simulink model "Dyn_Vol_Line"  (R2019b)
settings: Solver=ode4  StartTime=0.0  StopTime=5  FixedStep=0.0005  MaxStep=0.1  RelTol=1e-3  EnableMultiTasking=on
undefined symbols (not defined in the file): H2
libraries: Lib_Vol_pipeCd_TMATS x4, Lib_Vol_Volume_TMATS x4, Lib_Solve_ModelSource_TMATS x2, Lib_Vol_Valve_TMATS x2, Lib_Solve_IterNRSolverJC_TMATS x1, Lib_Vol_FlowChar_TMATS x1, Lib_Vol_FlowStart_TMATS x1, Lib_Vol_PropLookup_TMATS x1
settings Model: SimulationMode=rapid-accelerator  Creator=jwchapm2  LastModifiedBy=bhisma
settings DataIOCC: LimitDataPoints=on  SaveFormat=Array  ReturnWorkspaceOutputs=off
settings OptimizationCC: LifeSpan=inf
settings DebuggingCC: SFUnexpectedBacktrackingDiag=warning  SFNoUnconditionalDefaultTransitionDiag=warning  SFExecutionAtInitializationDiag=none  ArithmeticOperatorsInVariantConditions=warning
settings HardwareCC: ProdBitPerPointer=32  ProdBitPerSizeT=32  ProdBitPerPtrDiffT=32  ProdLargestAtomicFloat=None  ProdIntDivRoundTo=Undefined  ProdEndianess=Unspecified  ProdWordSize=32  ProdHWDeviceType=32-bit Generic
settings ModelReferenceCC: PropagateSignalLabelsOutOfModel=off
settings SFSimCC: SimUseLocalCustomCode=off  CustomCodeUndefinedFunction=UseInterfaceOnly
settings RTWCC: RTWUseLocalCustomCode=off
settings CodeAppCC: StateflowObjectComments=on
settings GRTTargetCC: TargetLangStandard=C89/C90 (ANSI)  GeneratePreprocessorConditionals=Disable all
settings ConfigComp: CovMetricSettings=dw  CovHtmlReporting=on  CovSaveCumulativeToWorkspaceVar=on  CovSaveSingleToWorkspaceVar=on  CovExternalEMLEnable=off

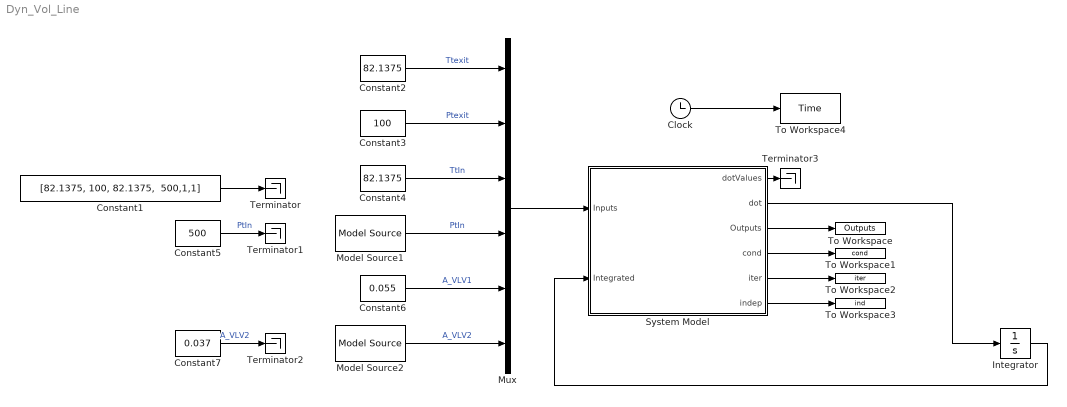
== system Dyn_Vol_Line ==
  Clock : Clock
  Constant1 : Constant  Value="[82.1375, 100, 82.1375,  500,1,1]"
  Constant2 : Constant  Value=82.1375
  Constant3 : Constant  Value=100
  Constant4 : Constant  Value=82.1375
  Constant5 : Constant  Value=500
  Constant6 : Constant  Value=0.055
  Constant7 : Constant  Value=0.037
  Integrator : Integrator  InitialCondition=[1.656, 47.38, 1.234, 52.46, 1.226, 52.55, 1.059, 54.12]
  Model Source1 : Lib_Solve_ModelSource_TMATS/Model Source  T_vec_M=[0 0.1 5]  input_array_M=[500 1000 50]
  Model Source2 : Lib_Solve_ModelSource_TMATS/Model Source  T_vec_M=[0 0.1 3 5]  input_array_M=[0.037 0.037 0 0 ]
  Mux : Mux  Inputs=6
  System Model : Subsystem
  Terminator{,1..3} (4 alike) : Terminator
  To Workspace : ToWorkspace  VariableName=Outputs  SampleTime=-1
      settings: Save2DSignal=2-D array (concatenate along first dimension)
  To Workspace1 : ToWorkspace  VariableName=cond  SampleTime=-1
      settings: Save2DSignal=2-D array (concatenate along first dimension)
  To Workspace2 : ToWorkspace  VariableName=iter  SampleTime=-1
      settings: Save2DSignal=2-D array (concatenate along first dimension)
  To Workspace3 : ToWorkspace  VariableName=ind  SampleTime=-1
      settings: Save2DSignal=2-D array (concatenate along first dimension)
  To Workspace4 : ToWorkspace  VariableName=Time  SampleTime=-1
      settings: Save2DSignal=2-D array (concatenate along first dimension)
  wires:
  Mux/1 -> System Model/1(Inputs)
  Integrator/1 -> System Model/2(Integrated)
  System Model/2(dot) -> Integrator/1
  Constant2/1 -> Mux/1  "Ttexit"
  Constant3/1 -> Mux/2  "Ptexit"
  Constant4/1 -> Mux/3  "TtIn"
  Model Source1/1 -> Mux/4  "PtIn"
  Constant6/1 -> Mux/5  "A_VLV1"
  Model Source2/1 -> Mux/6  "A_VLV2"
  System Model/3(Outputs) -> To Workspace/1
  System Model/4(cond) -> To Workspace1/1
  System Model/5(iter) -> To Workspace2/1
  System Model/6(indep) -> To Workspace3/1
  Clock/1 -> To Workspace4/1
  Constant1/1 -> Terminator/1
  Constant5/1 -> Terminator1/1  "PtIn"
  Constant7/1 -> Terminator2/1  "A_VLV2"
  System Model/1(dotValues) -> Terminator3/1

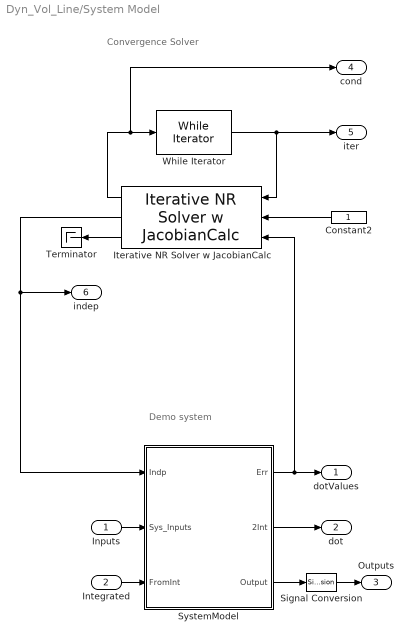
== system Dyn_Vol_Line/System Model ==
  note: Convergence Solver
  note: Demo system
  Inputs : Inport
  Integrated : Inport  Port=2
  Constant2 : Constant
  Iterative NR Solver w JacobianCalc : Lib_Solve_IterNRSolverJC_TMATS/Iterative NR Solver w JacobianCalc  SJac_Per_M=[0.05* ones(8,1)';-0.05* ones(8,1)']  SNR_IC_M=[453.3 98.05 303.8 98.05 301.2 98.05 251.1 98.05]  SNR_DX_M=1  SNR_Mx_M=100000  SNR_Mn_M=0.0001  SJacobianAttempts_M=50  Cond_Limits_M=0.00000001
  Signal Conversion : SignalConversion  OverrideOpt=off
  SystemModel : Subsystem  mask{Fluid=H2}
      mask prompts: Fluid "Fluid Type"
  Terminator : Terminator
  While Iterator : WhileIterator  MaxIters=200  WhileBlockType=do-while  ShowIterationPort=on
  dotValues : Outport
  dot : Outport  Port=2
  Outputs : Outport  Port=3
  cond : Outport  Port=4
  iter : Outport  Port=5
  indep : Outport  Port=6
  wires:
  Constant2/1 -> Iterative NR Solver w JacobianCalc/2
  Inputs/1 -> SystemModel/2(Sys_Inputs)
  SystemModel/1(Err) -> dotValues/1, Iterative NR Solver w JacobianCalc/3
  Iterative NR Solver w JacobianCalc/2 -> indep/1, SystemModel/1(Indp)
  SystemModel/2(2Int) -> dot/1
  Integrated/1 -> SystemModel/3(FromInt)
  Iterative NR Solver w JacobianCalc/1 -> cond/1, While Iterator/1
  While Iterator/1 -> iter/1, Iterative NR Solver w JacobianCalc/1
  Iterative NR Solver w JacobianCalc/3 -> Terminator/1
  SystemModel/3(Output) -> Signal Conversion/1
  Signal Conversion/1 -> Outputs/1

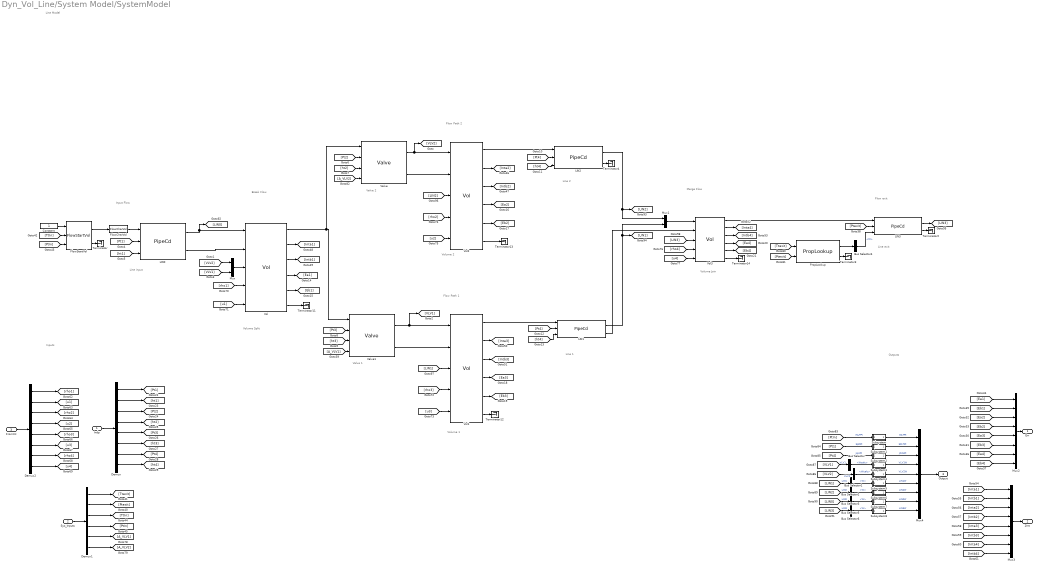
== system Dyn_Vol_Line/System Model/SystemModel ==
  note: Line Model
  note: Flow Path 2
  note: Flow Path 1
  note: Valve 2
  note: Valve 1
  note: Volume 1
  note: Line 1
  note: Volume 2
  note: Line 2
  note: Volume
      | Join
  note: Flow exit
  note: Merge
      | Flow
  note: Break
      | Flow
  note: Volume
      | Split
  note: Input Flow
  note: Line exit
  note: Inputs
  note: Outputs
  note: Line input
  Indp : Inport
  Sys_Inputs : Inport  Port=2
  FromInt : Inport  Port=3
  Bus Selector : BusSelector  OutputSignals=Wcalc
  Bus Selector1 : BusSelector  OutputSignals=Wcalc
  Bus Selector{2..3,5..6} (4 alike) : BusSelector  OutputSignals=W
  Bus Selector4 : BusSelector  OutputSignals=ht
  Constant : Constant
  Demux : Demux  Outputs=8
  Demux1 : Demux  Outputs=6
  Demux2 : Demux  Outputs=8
  FlowCharVol : Lib_Vol_FlowChar_TMATS/FlowCharVol  SystemSampleTime=-1
  FlowStartVol : Lib_Vol_FlowStart_TMATS/FlowStartVol  TtVec_M=Fluid.Vec.Tt  PtVec_M=Fluid.Vec.Pt  htVec_M=Fluid.Vec.ht  sVec_M=Fluid.Vec.s  htArray_M=Fluid.Array.ht  TtArray_M=Fluid.Array.Tt  sArray_M=Fluid.Array.s  rhoArray_M=Fluid.Array.rho  muArray_M=Fluid.Array.mu  CpArray_M=Fluid.Array.Cp  CvArray_M=Fluid.Array.Cv  CvArray_M_copy=Fluid.Array.u  Rval_M=Fluid.Array.R
  LIN0 : Lib_Vol_pipeCd_TMATS/PipeCd  Cd_M=0.5541  A_M=1  htVec_M=Fluid.Vec.ht  PtVec_M=Fluid.Vec.Pt  TtArray_M=Fluid.Array.Tt  rhoArray_M=Fluid.Array.rho
  LIN1 : Lib_Vol_pipeCd_TMATS/PipeCd  Cd_M=0.3859  A_M=1  htVec_M=Fluid.Vec.ht  PtVec_M=Fluid.Vec.Pt  TtArray_M=Fluid.Array.Tt  rhoArray_M=Fluid.Array.rho
  LIN2 : Lib_Vol_pipeCd_TMATS/PipeCd  Cd_M=0.2502  A_M=1  htVec_M=Fluid.Vec.ht  PtVec_M=Fluid.Vec.Pt  TtArray_M=Fluid.Array.Tt  rhoArray_M=Fluid.Array.rho
  LIN3 : Lib_Vol_pipeCd_TMATS/PipeCd  Cd_M=0.3985  A_M=1  htVec_M=Fluid.Vec.ht  PtVec_M=Fluid.Vec.Pt  TtArray_M=Fluid.Array.Tt  rhoArray_M=Fluid.Array.rho
  Mux : Mux  Inputs=2
  Mux1 : Mux  Inputs=2
  Mux2 : Mux  Inputs=8
  Mux3 : Mux  Inputs=8
  Mux4 : Mux  Inputs=9
  PropLookup : Lib_Vol_PropLookup_TMATS/PropLookup  case_M='ht'  propg_M=0  htg_M=0  htVec_M=Fluid.Vec.ht  PtVec_M=Fluid.Vec.Pt  TtVec_M=[-10000 10000]  sVec_M=[-10000 10000]  htArray_M=ones(2, length(Fluid.Vec.Pt))'  rhoArray_M=ones(length(Fluid.Vec.ht), length(Fluid.Vec.Pt))'  uArray_M=ones(length(Fluid.Vec.ht), length(Fluid.Vec.Pt))'  sArray_M=ones(length(Fluid.Vec.ht), length(Fluid.Vec.Pt))'  muArray_M=ones(length(Fluid.Vec.ht), length(Fluid.Vec.Pt))'  ThArray_M=Fluid.Array.Tt  CvArray_M=ones(length(Fluid.Vec.ht), length(Fluid.Vec.Pt))'  CpArray_M=ones(length(Fluid.Vec.ht), length(Fluid.Vec.Pt))'  kArray_M=ones(length(Fluid.Vec.ht), length(Fluid.Vec.Pt))'  TsArray_M=ones(2, length(Fluid.Vec.Pt))'  hsArray_M=ones(2, length(Fluid.Vec.Pt))'  Rval_M=0
  Subsystem : Subsystem
  Subsystem1 : Subsystem
  Subsystem2 : Subsystem
  Subsystem3 : Subsystem
  Subsystem4 : Subsystem
  Subsystem5 : Subsystem
  Subsystem6 : Subsystem
  Subsystem7 : Subsystem
  Subsystem8 : Subsystem
  Terminator{,2..4,11..14} (8 alike) : Terminator
  Valve : Lib_Vol_Valve_TMATS/Valve  Cd_M=3.4641  htVec_M=Fluid.Vec.ht  PtVec_M=Fluid.Vec.Pt  TtArray_M=Fluid.Array.Tt  rhoArray_M=Fluid.Array.rho
  Valve1 : Lib_Vol_Valve_TMATS/Valve  Cd_M=3.4641  htVec_M=Fluid.Vec.ht  PtVec_M=Fluid.Vec.Pt  TtArray_M=Fluid.Array.Tt  rhoArray_M=Fluid.Array.rho
  Vol : Lib_Vol_Volume_TMATS/Vol  volume_M=300  htVec_M=Fluid.Vec.ht  PtVec_M=Fluid.Vec.Pt  TtArray_M=Fluid.Array.Tt  uArray_M=Fluid.Array.u  rhoArray_M=Fluid.Array.rho
  Vol1 : Lib_Vol_Volume_TMATS/Vol  volume_M=1000  htVec_M=Fluid.Vec.ht  PtVec_M=Fluid.Vec.Pt  TtArray_M=Fluid.Array.Tt  uArray_M=Fluid.Array.u  rhoArray_M=Fluid.Array.rho
  Vol2 : Lib_Vol_Volume_TMATS/Vol  volume_M=500  htVec_M=Fluid.Vec.ht  PtVec_M=Fluid.Vec.Pt  TtArray_M=Fluid.Array.Tt  uArray_M=Fluid.Array.u  rhoArray_M=Fluid.Array.rho
  Vol3 : Lib_Vol_Volume_TMATS/Vol  volume_M=500  htVec_M=Fluid.Vec.ht  PtVec_M=Fluid.Vec.Pt  TtArray_M=Fluid.Array.Tt  uArray_M=Fluid.Array.u  rhoArray_M=Fluid.Array.rho
  Err : Outport
  2Int : Outport  Port=2
  Output : Outport  Port=3
  wires:
  Vol2/3 -> [Intb2]
  LIN3/2 -> Terminator2/1
  Bus Selector4/1 -> LIN3/3  "<ht>"
  [Ptexit] -> LIN3/2
  FlowStartVol/1 -> FlowCharVol/1
  FlowStartVol/2 -> Terminator/1
  LIN0/2 -> Vol/2
  Mux/1 -> Vol/3
  Valve/2 -> Vol2/2
  Valve1/2 -> Vol1/2
  Mux1/1 -> Vol3/1
  LIN1/2 -> Vol3/2
  [VLV2] -> Mux/1
  [VLV1] -> Mux/2
  [Pt1] -> LIN0/2
  [ht1] -> LIN0/3
  [ht2] -> Valve/3
  [Pt3] -> Valve1/2
  [ht3] -> Valve1/3
  [Pt4] -> LIN2/2
  [ht4] -> LIN2/3
  [ht4] -> LIN1/3
  Vol/4 -> [Ea1]
  Vol/5 -> [Eb1]
  Vol2/4 -> [Ea2]
  Vol2/5 -> [Eb2]
  Vol1/4 -> [Ea3]
  Vol1/5 -> [Eb3]
  Vol3/4 -> [Ea4]
  Vol3/5 -> [Eb4]
  Constant/1 -> FlowStartVol/1
  Mux2/1 -> Err/1
  Indp/1 -> Demux/1
  Vol2/2 -> [Inta2]
  [TtIn] -> FlowStartVol/2
  [Ea1] -> Mux2/1
  [Ea3] -> Mux2/5
  [Eb1] -> Mux2/2
  Demux/8 -> [ht4]
  Demux/5 -> [Pt3]
  Demux/2 -> [ht1]
  Demux/6 -> [ht3]
  [PtIn] -> FlowStartVol/3
  Demux/3 -> [Pt2]
  [Eb2] -> Mux2/4
  [Ea4] -> Mux2/7
  Demux/1 -> [Pt1]
  [Eb3] -> Mux2/6
  [Eb4] -> Mux2/8
  Demux/7 -> [Pt4]
  Demux/4 -> [ht2]
  [Ea2] -> Mux2/3
  Demux1/4 -> [PtIn]
  Demux1/3 -> [TtIn]
  Demux1/2 -> [Ptexit]
  Demux1/1 -> [Ttexit]
  Sys_Inputs/1 -> Demux1/1
  FlowCharVol/1 -> LIN0/1
  Vol1/1 -> LIN1/1
  Vol2/1 -> LIN2/1
  Vol3/1 -> LIN3/1
  LIN2/1 -> [LIN2], Mux1/1
  LIN1/1 -> [LIN1], Mux1/2
  LIN3/1 -> [LIN3]
  Valve/1 -> Vol2/1, [VLV2]
  Valve1/1 -> Vol1/1, [VLV1]
  LIN0/1 -> Vol/1, [LIN0]
  [Pt4] -> LIN1/2
  Vol/6 -> Terminator11/1
  Vol1/2 -> [Inta3]
  Vol1/3 -> [Intb3]
  Vol1/6 -> Terminator12/1
  Vol2/6 -> Terminator13/1
  Vol3/6 -> Terminator14/1
  Vol3/3 -> [Intb4]
  Vol3/2 -> [Inta4]
  Vol/2 -> [Inta1]
  Vol/3 -> [Intb1]
  [Inta3] -> Mux3/5
  [Intb2] -> Mux3/4
  [Intb3] -> Mux3/6
  [Inta4] -> Mux3/7
  [Inta2] -> Mux3/3
  [Intb1] -> Mux3/2
  [Intb4] -> Mux3/8
  [Inta1] -> Mux3/1
  Mux3/1 -> 2Int/1
  FromInt/1 -> Demux2/1
  Demux2/1 -> [rho1]
  Demux2/2 -> [u1]
  Demux2/3 -> [rho2]
  Demux2/4 -> [u2]
  Demux2/5 -> [rho3]
  Demux2/6 -> [u3]
  Demux2/7 -> [rho4]
  Demux2/8 -> [u4]
  [u1] -> Vol/5
  [rho1] -> Vol/4
  [rho3] -> Vol1/4
  [u3] -> Vol1/5
  [rho2] -> Vol2/4
  [u2] -> Vol2/5
  [rho4] -> Vol3/4
  [u4] -> Vol3/5
  Demux1/5 -> [A_VLV1]
  Demux1/6 -> [A_VLV2]
  [Ttexit] -> PropLookup/1
  [Ptexit] -> PropLookup/2
  PropLookup/1 -> Bus Selector4/1
  PropLookup/2 -> Terminator3/1
  [A_VLV2] -> Valve/4
  [A_VLV1] -> Valve1/4
  [VLV1] -> Bus Selector/1  "VLV1"
  [VLV2] -> Bus Selector1/1  "VLV2"
  [LIN1] -> Bus Selector2/1  "LIN1"
  [LIN2] -> Bus Selector3/1  "LIN2"
  [LIN0] -> Bus Selector5/1  "LIN0"
  [LIN3] -> Bus Selector6/1  "LIN3"
  [PtIn] -> Subsystem/1(In1)  "INLTPt"
  [Pt1] -> Subsystem1/1(In1)  "SpltPt"
  [Pt4] -> Subsystem2/1(In1)  "JoinPt"
  Bus Selector/1 -> Subsystem3/1(In1)  "<Wcalc>"
  Bus Selector1/1 -> Subsystem4/1(In1)  "<Wcalc>"
  Bus Selector2/1 -> Subsystem5/1(In1)  "<W>"
  Bus Selector3/1 -> Subsystem6/1(In1)  "<W>"
  Bus Selector5/1 -> Subsystem7/1(In1)  "<W>"
  Bus Selector6/1 -> Subsystem8/1(In1)  "<W>"
  Mux4/1 -> Output/1
  Subsystem/1(Out1) -> Mux4/1  "INLTPt"
  Subsystem1/1(Out1) -> Mux4/2  "SPLTPt"
  Subsystem2/1(Out1) -> Mux4/3  "JOINPt"
  Subsystem3/1(Out1) -> Mux4/4  "VLV1W"
  Subsystem4/1(Out1) -> Mux4/5  "VLV2W"
  Subsystem5/1(Out1) -> Mux4/6  "LIN1W"
  Subsystem6/1(Out1) -> Mux4/7  "LIN2W"
  Subsystem7/1(Out1) -> Mux4/8  "LIN0W"
  Subsystem8/1(Out1) -> Mux4/9  "LIN3W"
  LIN2/2 -> Terminator4/1
  [LIN2] -> Vol2/3
  [LIN1] -> Vol1/3
  [LIN3] -> Vol3/3
  Vol/1 -> Valve1/1, Valve/1
  [Pt2] -> Valve/2

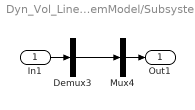
== system Dyn_Vol_Line/System Model/SystemModel/Subsystem ==
  In1 : Inport
  Demux3 : Demux  Outputs=1
  Mux4 : Mux  Inputs=1
  Out1 : Outport
  wires:
  Demux3/1 -> Mux4/1
  In1/1 -> Demux3/1
  Mux4/1 -> Out1/1

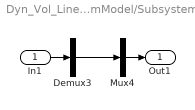
== system Dyn_Vol_Line/System Model/SystemModel/Subsystem1 ==
  In1 : Inport
  Demux3 : Demux  Outputs=1
  Mux4 : Mux  Inputs=1
  Out1 : Outport
  wires:
  Mux4/1 -> Out1/1
  In1/1 -> Demux3/1
  Demux3/1 -> Mux4/1

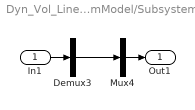
== system Dyn_Vol_Line/System Model/SystemModel/Subsystem2 ==
  In1 : Inport
  Demux3 : Demux  Outputs=1
  Mux4 : Mux  Inputs=1
  Out1 : Outport
  wires:
  Demux3/1 -> Mux4/1
  In1/1 -> Demux3/1
  Mux4/1 -> Out1/1

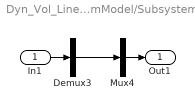
== system Dyn_Vol_Line/System Model/SystemModel/Subsystem3 ==
  In1 : Inport
  Demux3 : Demux  Outputs=1
  Mux4 : Mux  Inputs=1
  Out1 : Outport
  wires:
  Mux4/1 -> Out1/1
  In1/1 -> Demux3/1
  Demux3/1 -> Mux4/1

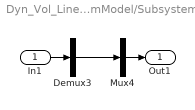
== system Dyn_Vol_Line/System Model/SystemModel/Subsystem4 ==
  In1 : Inport
  Demux3 : Demux  Outputs=1
  Mux4 : Mux  Inputs=1
  Out1 : Outport
  wires:
  Demux3/1 -> Mux4/1
  In1/1 -> Demux3/1
  Mux4/1 -> Out1/1

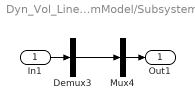
== system Dyn_Vol_Line/System Model/SystemModel/Subsystem5 ==
  In1 : Inport
  Demux3 : Demux  Outputs=1
  Mux4 : Mux  Inputs=1
  Out1 : Outport
  wires:
  Mux4/1 -> Out1/1
  In1/1 -> Demux3/1
  Demux3/1 -> Mux4/1

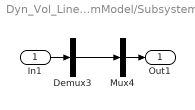
== system Dyn_Vol_Line/System Model/SystemModel/Subsystem6 ==
  In1 : Inport
  Demux3 : Demux  Outputs=1
  Mux4 : Mux  Inputs=1
  Out1 : Outport
  wires:
  Demux3/1 -> Mux4/1
  In1/1 -> Demux3/1
  Mux4/1 -> Out1/1

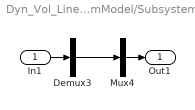
== system Dyn_Vol_Line/System Model/SystemModel/Subsystem7 ==
  In1 : Inport
  Demux3 : Demux  Outputs=1
  Mux4 : Mux  Inputs=1
  Out1 : Outport
  wires:
  Mux4/1 -> Out1/1
  In1/1 -> Demux3/1
  Demux3/1 -> Mux4/1

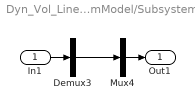
== system Dyn_Vol_Line/System Model/SystemModel/Subsystem8 ==
  In1 : Inport
  Demux3 : Demux  Outputs=1
  Mux4 : Mux  Inputs=1
  Out1 : Outport
  wires:
  Demux3/1 -> Mux4/1
  In1/1 -> Demux3/1
  Mux4/1 -> Out1/1
